simulink model "Asyncronous_model"  (R2018b)
settings: Solver=VariableStepAuto  StartTime=0.0  StopTime=0.2  FixedStep=sampletime  MaxStep=1e-4  RelTol=1e-5
settings Model: Creator=Lac  LastModifiedBy=Lac

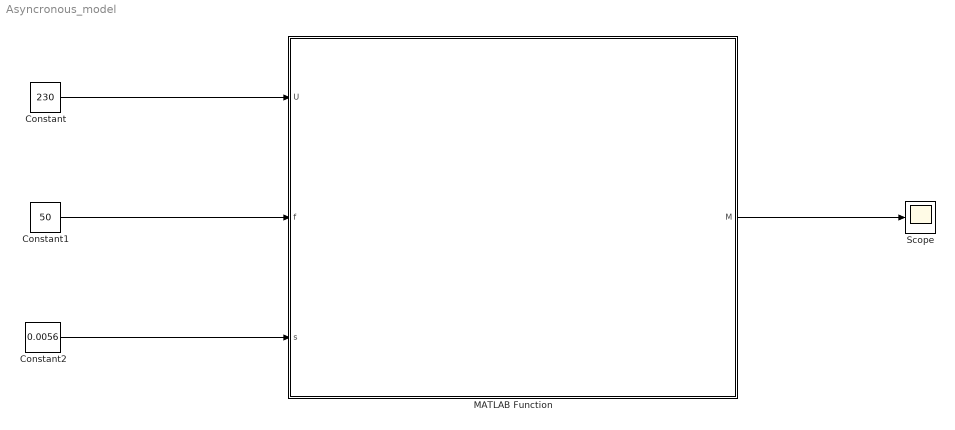
== system Asyncronous_model ==
  Constant : Constant  Value=230
  Constant1 : Constant  Value=50
  Constant2 : Constant  Value=0.0056
  MATLAB Function : MATLAB Function  TreatAsAtomicUnit=on
  Scope : Scope
  wires:
  MATLAB Function/1(M) -> Scope/1
  Constant2/1 -> MATLAB Function/3(s)
  Constant1/1 -> MATLAB Function/2(f)
  Constant/1 -> MATLAB Function/1(U)

== matlab function Asyncronous_model/MATLAB Function ==
  data: M output; U input; f input; s input
function M = Motor(U,f,s)
cosfi=0.85
p=2

Lm=0.0080335
Xm=Lm*2*pi*f
L2=0.0002406
R2=0.0072
X2=L2*2*pi*f
Zn=abs(R2+(1i*X2)+((1/(1i*Xm))+(1/(R2+(1i*X2)+(R2*((1-s)/s)))))^(-1))

I1_abs=U/Zn;
I1=I1_abs*(cosfi-(1i*sin(acos(cosfi))))
Im=U/(1i*Xm)
I2=I1-Im
I2_abs=abs(I2)
Rm=R2*((1-s)/s)
Pmech=((abs(I2))^2)*3*Rm
n=((60*f)/(p/2))*(1-s)
omega=(n/60)*2*pi
M=Pmech/omega
